simulink model "Tape_Drive_PID"  (R2025b)
settings: Solver=VariableStepAuto  StartTime=0.0  StopTime=10.0  RelTol=1e-3
values from neighbouring files (symbols this model uses):
  B = 20    [System_Parameters.m]
  B1 = 1e-2    (= 0.01)    [System_Parameters.m]
  B2 = 2e-2    (= 0.02)    [System_Parameters.m]
  J1 = 5e-5    (= 5e-05)    [System_Parameters.m]
  J2 = 2e-5    (= 2e-05)    [System_Parameters.m]
  K = 2e4    (= 20000)    [System_Parameters.m]
  Kd = 0.025    [System_Parameters.m]
  Ki = 6250    [System_Parameters.m]
  Kp = 50    [System_Parameters.m]
  Kt = 3e-2    (= 0.03)    [System_Parameters.m]
  r1 = 2e-2    (= 0.02)    [System_Parameters.m]
  r2 = 2e-2    (= 0.02)    [System_Parameters.m]
libraries: slpidlib x1
settings Model: Creator=AsusIran  LastModifiedBy=AsusIran

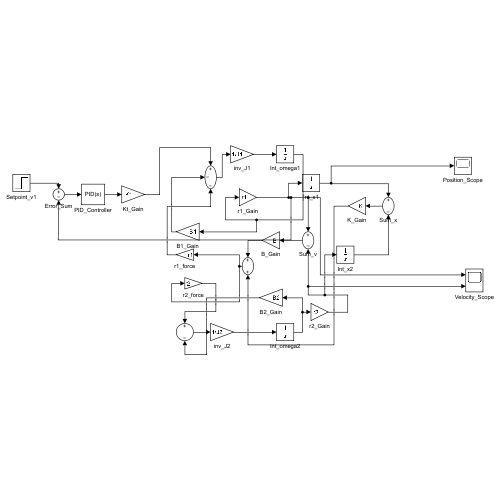
[thumbnail: Simulink's stored preview of the top-level diagram]
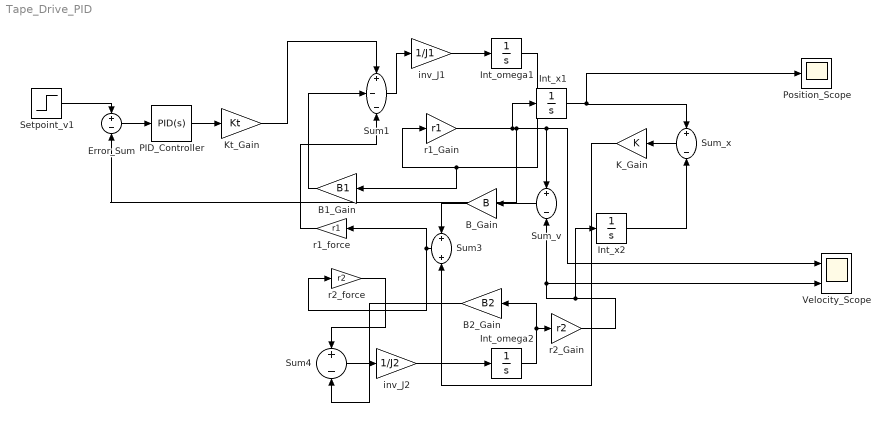
== system Tape_Drive_PID ==
  B1_Gain : Gain  Gain=B1
  B2_Gain : Gain  Gain=B2
  B_Gain : Gain  Gain=B
  Error_Sum : Sum  Inputs=+-
  Int_omega1 : Integrator
  Int_omega2 : Integrator
  Int_x1 : Integrator
  Int_x2 : Integrator
  K_Gain : Gain  Gain=K
  Kt_Gain : Gain  Gain=Kt
  PID_Controller : slpidlib/PID Controller  Controller=PID  Form=Parallel  TimeDomain=Continuous-time  UseExternalTs=off  SampleTime=-1  IntegratorMethod=Forward Euler  FilterMethod=Forward Euler  ControllerParametersSource=internal  P=Kp  I=Ki  UseKiTs=off  D=Kd  UseExternalDerivativeSource=off  N=100  UseFilter=on  TunerSelectOption=Transfer Function Based (PID Tuner App)  InitialConditionSource=internal  InitialConditionForIntegrator=0  InitialConditionForFilter=0  DifferentiatorICPrevScaledInput=0  ExternalReset=none  TrackingMode=off  Kt=1  LimitOutput=off  SatLimitsSource=internal  UpperSaturationLimit=inf  LowerSaturationLimit=-inf  LinearizeAsGain=on  AntiWindupMode=none  Kb=1  LimitIntegrator=off  UpperIntegratorSaturationLimit=inf  LowerIntegratorSaturationLimit=-inf  POutMin=[]  POutMax=[]  IOutMin=[]  IOutMax=[]  DOutMin=[]  DOutMax=[]  NOutMin=[]  NOutMax=[]  SumOutMin=[]  SumOutMax=[]  SaturationOutMin=[]  SaturationOutMax=[]  PParamMin=[]  PParamMax=[]  IParamMin=[]  IParamMax=[]  DParamMin=[]  DParamMax=[]  NParamMin=[]  NParamMax=[]  KbParamMin=[]  KbParamMax=[]  KtParamMin=[]  KtParamMax=[]  KbOutMin=[]  KbOutMax=[]  KtOutMin=[]  KtOutMax=[]  IntegratorOutMin=[]  IntegratorOutMax=[]  FilterOutMin=[]  FilterOutMax=[]  SumI1OutMin=[]  SumI1OutMax=[]  SumI2OutMin=[]  SumI2OutMax=[]  SumI3OutMin=[]  SumI3OutMax=[]  SumI4OutMin=[]  SumI4OutMax=[]  SumDOutMin=[]  SumDOutMax=[]  DifferentiatorOutMin=[]  DifferentiatorOutMax=[]  FilterDiffOutCoefMin=[]  FilterDiffOutCoefMax=[]  ReciprocalOutMin=[]  ReciprocalOutMax=[]  SumDenOutMin=[]  SumDenOutMax=[]  SumNumOutMin=[]  SumNumOutMax=[]  DivideOutMin=[]  DivideOutMax=[]  UdiffTsProdOutMin=[]  UdiffTsProdOutMax=[]  NTsProdOutMin=[]  NTsProdOutMax=[]  UintegralTsProdOutMin=[]  UintegralTsProdOutMax=[]  UngainTsProdOutMin=[]  UngainTsProdOutMax=[]  ClampingZeroOutDataTypeStr=Inherit: Inherit via back propagation  ClampingZeroOutMin=[]  ClampingZeroOutMax=[]  FilterDenConstantOutDataTypeStr=Inherit: Inherit via back propagation  FilterDenConstantOutMin=[]  FilterDenConstantOutMax=[]  PCopyOutDataTypeStr=Inherit: Inherit via back propagation  PCopyOutMin=[]  PCopyOutMax=[]  NCopyOutDataTypeStr=Inherit: Inherit via back propagation  NCopyOutMin=[]  NCopyOutMax=[]  IntegratorContinuousStateAttributes=''  IntegratorStateMustResolveToSignalObject=off  IntegratorRTWStateStorageClass=Auto  FilterContinuousStateAttributes=''  FilterStateMustResolveToSignalObject=off  FilterRTWStateStorageClass=Auto  ParallelPVariant=InternalParameters  IdealPVariant=Disabled  IVariant=InternalParameters  DVariant=InternalParameters  IntegratorVariant=Continuous  SatVariant=Disabled  AWVariant=Passthrough  PCopyVariant=Disabled  TRVariant=Disabled  FdbkBlocksVariant=Forward  IdealPFdbkVariant=Disabled  SatFdbkVariant=Disabled  DerivativeFilterVariant=ContFilter  NVariant=InternalParameters  NCopyVariant=Disabled  FilterICVariant=InternalICsFilter  IntegratorICVariant=InternalICs  ExternalResetVariant=Disabled  TRSumVariant=Passthrough  SumFdbkVariant=Disabled  SumVariant=Sum_PID  TsampFilterVariant=InternalTs  TsampNgainVariant=Passthrough  TsampIntegralVariant=Disabled_SignalSpec  ExternalSaturationOutDataTypeStr=Inherit: Same as second input  DerivativeSourceVariant=ErrorSignal  PreIntVariant=InternalPreInt
  Position_Scope : Scope
      settings: ActiveDisplayYMinimum=-1.2475138256204417  ActiveDisplayYMaximum=11.227624430583976
  Setpoint_v1 : Step  Time=0  SampleTime=0
  Sum1 : Sum  Inputs=+--
  Sum3 : Sum
  Sum4 : Sum  Inputs=+-
  Sum_v : Sum  Inputs=+-
  Sum_x : Sum  Inputs=+-
  Velocity_Scope : Scope  NumInputPorts=2
      settings: ActiveDisplayYMinimum=-0.1251379051784455  ActiveDisplayYMaximum=1.1262411466060098
  inv_J1 : Gain  Gain=1/J1
  inv_J2 : Gain  Gain=1/J2
  r1_Gain : Gain  Gain=r1
  r1_force : Gain  Gain=r1
  r2_Gain : Gain  Gain=r2
  r2_force : Gain  Gain=r2
  wires:
  Setpoint_v1/1 -> Error_Sum/1
  Error_Sum/1 -> PID_Controller/1
  PID_Controller/1 -> Kt_Gain/1
  Kt_Gain/1 -> Sum1/1
  Sum1/1 -> inv_J1/1
  inv_J1/1 -> Int_omega1/1
  Int_omega1/1 -> r1_Gain/1, B1_Gain/1
  B1_Gain/1 -> Sum1/2
  r1_Gain/1 -> Sum_v/1, Velocity_Scope/1, Error_Sum/2, Int_x1/1
  Int_x1/1 -> Sum_x/1, Position_Scope/1
  Sum4/1 -> inv_J2/1
  inv_J2/1 -> Int_omega2/1
  Int_omega2/1 -> B2_Gain/1, r2_Gain/1
  B2_Gain/1 -> Sum4/2
  r2_Gain/1 -> Velocity_Scope/2, Sum_v/2, Int_x2/1
  Int_x2/1 -> Sum_x/2
  Sum_v/1 -> B_Gain/1
  B_Gain/1 -> Sum3/1
  Sum_x/1 -> K_Gain/1
  K_Gain/1 -> Sum3/2
  Sum3/1 -> r1_force/1, r2_force/1
  r1_force/1 -> Sum1/3
  r2_force/1 -> Sum4/1
